simulink model "LAB2_1_PID_2024"  (R2024b)
settings: Solver=FixedStepDiscrete  StartTime=0.0  StopTime=10  FixedStep=T  RelTol=1e-3
values from neighbouring files (symbols this model uses):
  Dd = Dd_options(method_choice,:)    [LAB2_1_PID.m]
  Kw = 5/0.15    (= 33.3333333333)    [LAB2_1_PID.m]
  method_choice = input('Choose discretization method (1 = B. Euler, 2 = F. Euler, 3 = Tustin, 4 = Exact): ')    [LAB2_1_PID.m]
  Nd = Nd_options(method_choice,:)    [LAB2_1_PID.m]
  step_amplitude = 360    [LAB2_1_PID.m]
  T = input('Select sample time (0.001, 0.01, 0.05) [s]: ')    [LAB2_1_PID.m]    (also in prova_plot.m = 0.001)
undefined symbols (not defined in the file or in its folder): daq, den_Hi, Di_exact, DiscIntNeverNeededParam, Kd, Ki, Kp, mot, National_Instruments, Ni_exact, num_Hi, PCI, pulse2deg, sens
libraries: sldrtlib x3
settings Model: SimulationMode=external  ExtModeTrigDuration=100001  Creator=delpratogi  LastModifiedBy=Gioele
settings DataIOCC: ReturnWorkspaceOutputs=off
settings HardwareCC: ProdBitPerLong=64  ProdHWDeviceType=Intel->x86-64 (Linux 64)
settings RTWCC: Description=Simulink Desktop Real-Time  SystemTargetFile=sldrt.tlc  TemplateMakefile=sldrt.tmf  RTWCompilerOptimization=on
settings CodeAppCC: MaxIdLength=95
settings SimulinkDesktopRealTimeCC: TargetLibSuffix=_sldrt.a  TargetPreCompLibLocation=C:\Program Files\MATLAB\R2025b\toolbox\sldrt\lib\win64  ParMdlRefBuildCompliant=on  SubcomponentCodeInterfacePackaging=Reusable function  SupportVariableSizeSignals=off
settings ConfigComp: CovBoundaryAbsTol=1.0e-5

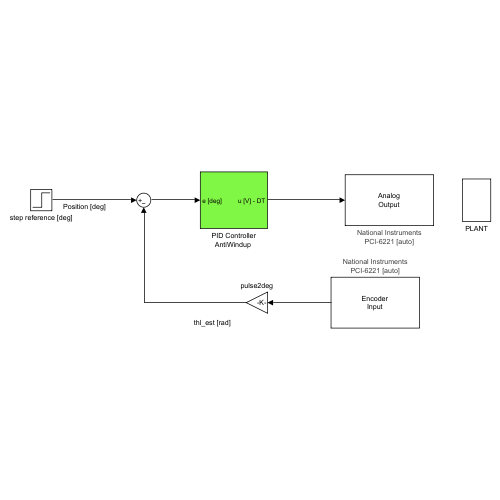
[thumbnail: Simulink's stored preview of the top-level diagram]
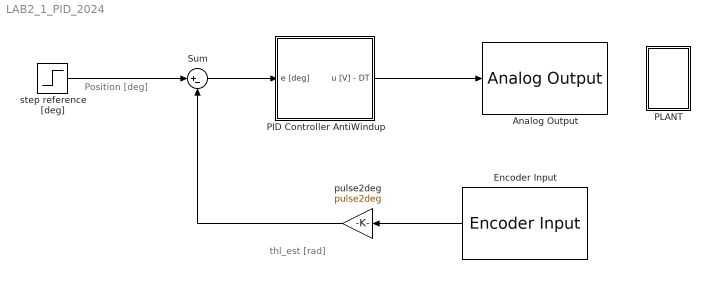
== system LAB2_1_PID_2024 ==
  note: Position [deg]
  note: thl_est [rad]
  Analog Output : sldrtlib/Analog Output  SampleTime=0.001  MaxMissedTicks=10  ShowMissedTicks=off  YieldWhenWaiting=off  DrvName=National_Instruments/PCI-6221  DrvAddress=4294967295  DrvOptions=[0 0 0 2 0]  Channels=1  RangeMode=1  VoltRange=1  InitialValue=0  FinalValue=0
      settings: AttributesFormatString=National Instruments\nPCI-6221 [auto]
  Encoder Input : sldrtlib/Encoder Input  SampleTime=0.001  MaxMissedTicks=10  ShowMissedTicks=off  YieldWhenWaiting=off  DrvName=National_Instruments/PCI-6221  DrvAddress=4294967295  DrvOptions=[0 0 0 2 0]  Channels=1  QuadMode=3  IndexPulse=1  InputFilter=Inf  DataType=1
      settings: AttributesFormatString=National Instruments\nPCI-6221 [auto]
  "PID Controller AntiWindup " : Subsystem
  PLANT : Subsystem
  Sum : Sum  Inputs=|+-
  pulse2deg : Gain  Gain=pulse2deg
  step reference [deg] : Step  After=step_amplitude  SampleTime=T
  wires:
  pulse2deg/1 -> Sum/2
  Sum/1 -> "PID Controller AntiWindup "/1("e [deg] ")
  "PID Controller AntiWindup "/1(u [V] - DT) -> Analog Output/1
  step reference [deg]/1 -> Sum/1
  Encoder Input/1 -> pulse2deg/1

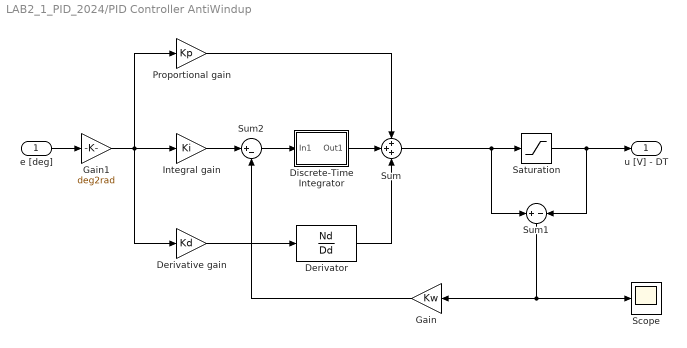
== system LAB2_1_PID_2024/PID Controller AntiWindup  ==
  "e [deg] " : Inport
  Derivative gain : Gain  Gain=Kd
  "Derivator " : DiscreteTransferFcn  Numerator=Nd  Denominator=Dd
  Discrete-Time Integrator : Subsystem
  Gain : Gain  Gain=Kw
  Gain1 : Gain  Gain=deg2rad
  "Integral gain " : Gain  Gain=Ki
  Proportional gain : Gain  Gain=Kp
  Saturation : Saturate  UpperLimit=daq.dac.fs  LowerLimit=-daq.dac.fs
  Scope : Scope
  Sum : Sum  Inputs=+++
  Sum1 : Sum  Inputs=+|-
  Sum2 : Sum  Inputs=|+-
  u [V] - DT : Outport
  wires:
  "Derivator "/1 -> Sum/3
  "e [deg] "/1 -> Gain1/1
  Proportional gain/1 -> Sum/1
  Derivative gain/1 -> "Derivator "/1
  Saturation/1 -> Sum1/2, u [V] - DT/1
  Sum1/1 -> Gain/1, Scope/1
  "Integral gain "/1 -> Sum2/1
  Gain/1 -> Sum2/2
  Sum/1 -> Sum1/1, Saturation/1
  Sum2/1 -> Discrete-Time Integrator/1(In1)
  Gain1/1 -> Proportional gain/1, Derivative gain/1, "Integral gain "/1
  Discrete-Time Integrator/1(Out1) -> Sum/2

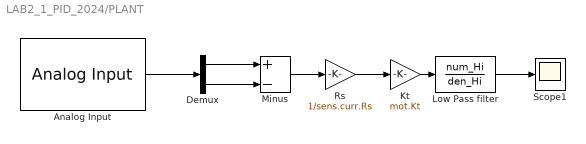
== system LAB2_1_PID_2024/PLANT ==
  Analog Input : sldrtlib/Analog Input  SampleTime=0.001  MaxMissedTicks=10  ShowMissedTicks=off  YieldWhenWaiting=off  DrvName=National_Instruments/PCI-6221  DrvAddress=4294967295  DrvOptions=[0 0 0 2 0]  Channels=[1,2]  RangeMode=1  VoltRange=1  DataType=1
      settings: AttributesFormatString=National Instruments\nPCI-6221 [auto]
  Demux : Demux  Outputs=2
  Kt : Gain  Gain=mot.Kt
  Low Pass filter : TransferFcn  Numerator=num_Hi  Denominator=den_Hi
  Minus : Sum  Inputs=+-
  Rs : Gain  Gain=1/sens.curr.Rs
  Scope1 : Scope
  wires:
  Low Pass filter/1 -> Scope1/1
  Demux/1 -> Minus/1
  Minus/1 -> Rs/1
  Analog Input/1 -> Demux/1
  Kt/1 -> Low Pass filter/1
  Demux/2 -> Minus/2
  Rs/1 -> Kt/1

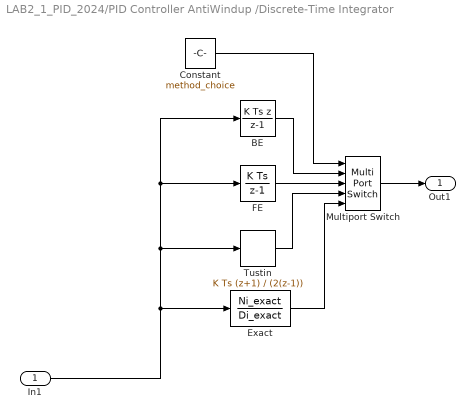
== system LAB2_1_PID_2024/PID Controller AntiWindup /Discrete-Time Integrator ==
  In1 : Inport
  BE : DiscreteIntegrator  IntegratorMethod=Integration: Backward Euler  SampleTime=T  ICPrevOutput=DiscIntNeverNeededParam  ICPrevScaledInput=DiscIntNeverNeededParam
  Constant : Constant  Value=method_choice
  Exact : DiscreteTransferFcn  Numerator=Ni_exact  Denominator=Di_exact
  "FE " : DiscreteIntegrator  SampleTime=T  ICPrevOutput=DiscIntNeverNeededParam  ICPrevScaledInput=DiscIntNeverNeededParam
  Multiport Switch : MultiPortSwitch  Inputs=4  SaturateOnIntegerOverflow=off  InputSameDT=off
  Tustin : DiscreteIntegrator  IntegratorMethod=Integration: Trapezoidal  SampleTime=T  ICPrevOutput=DiscIntNeverNeededParam  ICPrevScaledInput=DiscIntNeverNeededParam
  Out1 : Outport
  wires:
  In1/1 -> Exact/1, BE/1, "FE "/1, Tustin/1
  Constant/1 -> Multiport Switch/1
  "FE "/1 -> Multiport Switch/3
  BE/1 -> Multiport Switch/2
  Tustin/1 -> Multiport Switch/4
  Multiport Switch/1 -> Out1/1
  Exact/1 -> Multiport Switch/5
